simulink model "feedback_sys"  (R2017a)
settings: Solver=VariableStepAuto  StartTime=0.0  StopTime=10.0  RelTol=1e-3
settings Model: Creator=Priyesh  LastModifiedBy=Priyesh

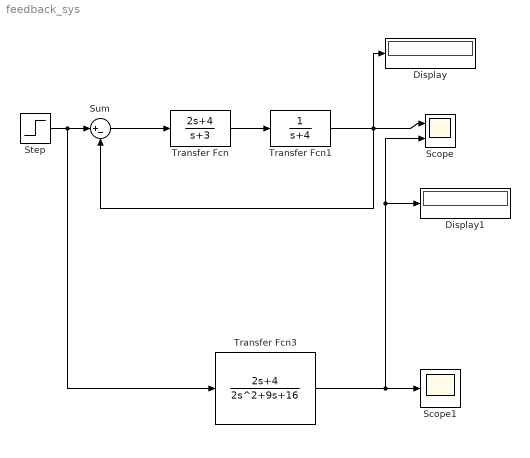
== system feedback_sys ==
  Display : Display
  Display1 : Display
  Scope : Scope  NumInputPorts=2
  Scope1 : Scope
  Step : Step  SampleTime=0
  Sum : Sum  Inputs=|+-
  Transfer Fcn : TransferFcn  Numerator=[2 4]  Denominator=[1 3]
  Transfer Fcn1 : TransferFcn  Denominator=[1 4]
  Transfer Fcn3 : TransferFcn  Numerator=[2 4]  Denominator=[2 9 16]
  wires:
  Transfer Fcn/1 -> Transfer Fcn1/1
  Sum/1 -> Transfer Fcn/1
  Step/1 -> Transfer Fcn3/1, Sum/1
  Transfer Fcn3/1 -> Display1/1, Scope/2, Scope1/1
  Transfer Fcn1/1 -> Display/1, Sum/2, Scope/1
